simulink model "BitwiseAnd"  (R2014a)
settings: Solver=ode45  StartTime=0.0  StopTime=10.0  RelTol=1e-3
libraries: hdlsllib x17
settings Model: Creator=you.r  LastModifiedBy=you.r

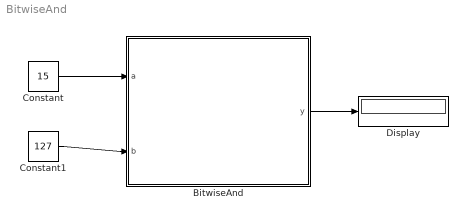
== system BitwiseAnd ==
  BitwiseAnd : Subsystem
  Constant : Constant  Value=15  OutDataTypeStr=uint8  SampleTime=1
  Constant1 : Constant  Value=127  OutDataTypeStr=uint8  SampleTime=-1
  Display : Display
  wires:
  Constant/1 -> BitwiseAnd/1(a)
  Constant1/1 -> BitwiseAnd/2(b)
  BitwiseAnd/1(y) -> Display/1

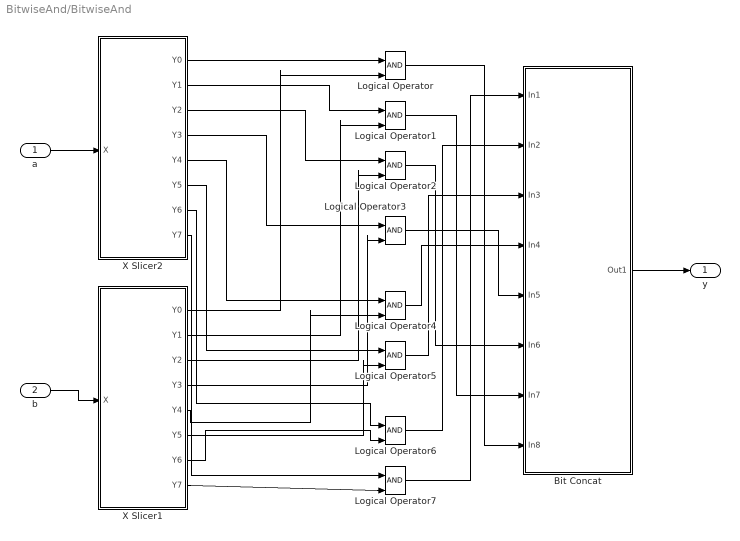
== system BitwiseAnd/BitwiseAnd ==
  a : Inport  OutDataTypeStr=uint8  SampleTime=1
  b : Inport  Port=2  OutDataTypeStr=uint8  SampleTime=1
  Bit Concat : Subsystem
  Logical Operator{,1..7} (8 alike) : Logic  IconShape=distinctive  AllPortsSameDT=off  OutDataTypeStr=boolean  SampleTime=1
  X Slicer1 : Subsystem
  X Slicer2 : Subsystem
  y : Outport  SampleTime=1
  wires:
  b/1 -> X Slicer1/1(X)
  a/1 -> X Slicer2/1(X)
  Logical Operator2/1 -> Bit Concat/6(In6)
  Logical Operator4/1 -> Bit Concat/4(In4)
  Logical Operator7/1 -> Bit Concat/1(In1)
  Logical Operator/1 -> Bit Concat/8(In8)
  Logical Operator1/1 -> Bit Concat/7(In7)
  Logical Operator6/1 -> Bit Concat/2(In2)
  Logical Operator5/1 -> Bit Concat/3(In3)
  Logical Operator3/1 -> Bit Concat/5(In5)
  X Slicer1/8(Y7) -> Logical Operator7/2
  X Slicer1/5(Y4) -> Logical Operator4/2
  X Slicer2/4(Y3) -> Logical Operator3/1
  X Slicer2/8(Y7) -> Logical Operator7/1
  X Slicer2/3(Y2) -> Logical Operator2/1
  X Slicer2/6(Y5) -> Logical Operator5/1
  X Slicer2/2(Y1) -> Logical Operator1/1
  X Slicer1/3(Y2) -> Logical Operator2/2
  X Slicer1/2(Y1) -> Logical Operator1/2
  X Slicer1/7(Y6) -> Logical Operator6/2
  X Slicer2/7(Y6) -> Logical Operator6/1
  X Slicer2/5(Y4) -> Logical Operator4/1
  X Slicer1/1(Y0) -> Logical Operator/2
  X Slicer2/1(Y0) -> Logical Operator/1
  X Slicer1/6(Y5) -> Logical Operator5/2
  X Slicer1/4(Y3) -> Logical Operator3/2
  Bit Concat/1(Out1) -> y/1

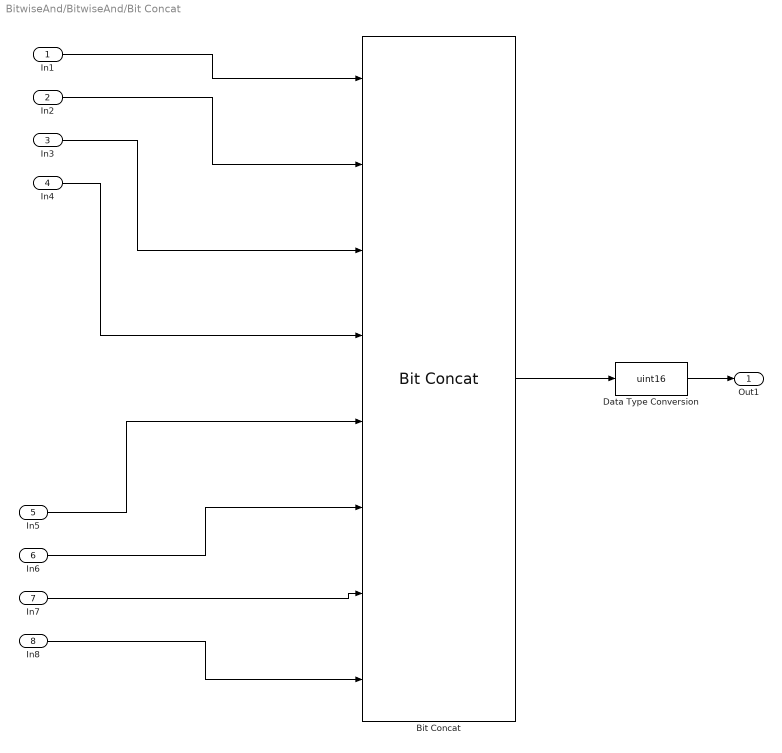
== system BitwiseAnd/BitwiseAnd/Bit Concat ==
  In1 : Inport
  In2 : Inport  Port=2
  In3 : Inport  Port=3
  In4 : Inport  Port=4
  In5 : Inport  Port=5
  In6 : Inport  Port=6
  In7 : Inport  Port=7
  In8 : Inport  Port=8
  Bit Concat : hdlsllib/HDL Operations/Bit Concat  numInputs=8
  Data Type Conversion : DataTypeConversion  OutDataTypeStr=uint16
  Out1 : Outport
  wires:
  Data Type Conversion/1 -> Out1/1
  Bit Concat/1 -> Data Type Conversion/1
  In7/1 -> Bit Concat/7
  In1/1 -> Bit Concat/1
  In8/1 -> Bit Concat/8
  In6/1 -> Bit Concat/6
  In2/1 -> Bit Concat/2
  In5/1 -> Bit Concat/5
  In3/1 -> Bit Concat/3
  In4/1 -> Bit Concat/4

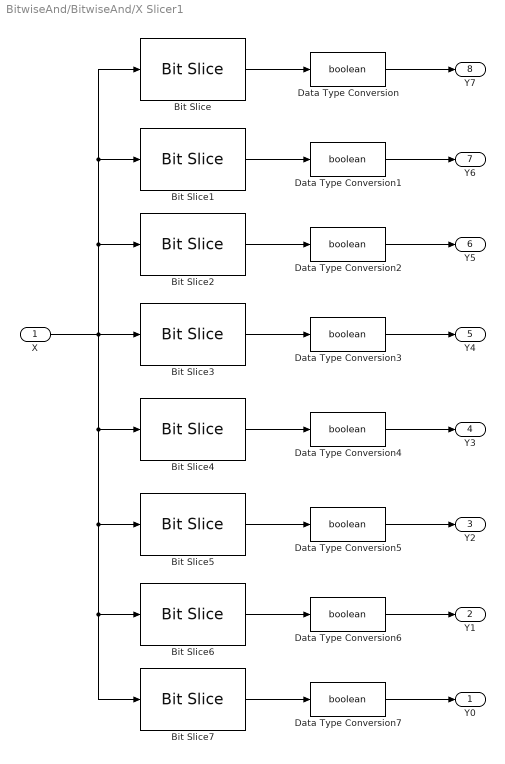
== system BitwiseAnd/BitwiseAnd/X Slicer1 ==
  X : Inport  OutDataTypeStr=uint8  SampleTime=1
  Bit Slice : hdlsllib/HDL Operations/Bit Slice  lidx=7  ridx=7
  Bit Slice1 : hdlsllib/HDL Operations/Bit Slice  lidx=6  ridx=6
  Bit Slice2 : hdlsllib/HDL Operations/Bit Slice  lidx=5  ridx=5
  Bit Slice3 : hdlsllib/HDL Operations/Bit Slice  lidx=4  ridx=4
  Bit Slice4 : hdlsllib/HDL Operations/Bit Slice  lidx=3  ridx=3
  Bit Slice5 : hdlsllib/HDL Operations/Bit Slice  lidx=2  ridx=2
  Bit Slice6 : hdlsllib/HDL Operations/Bit Slice  lidx=1  ridx=1
  Bit Slice7 : hdlsllib/HDL Operations/Bit Slice  lidx=0  ridx=0
  Data Type Conversion{,1..7} (8 alike) : DataTypeConversion  OutDataTypeStr=boolean
  Y0 : Outport  OutDataTypeStr=boolean  SampleTime=1
  Y1 : Outport  Port=2  OutDataTypeStr=boolean  SampleTime=1
  Y2 : Outport  Port=3  OutDataTypeStr=boolean  SampleTime=1
  Y3 : Outport  Port=4  OutDataTypeStr=boolean  SampleTime=1
  Y4 : Outport  Port=5  OutDataTypeStr=boolean  SampleTime=1
  Y5 : Outport  Port=6  OutDataTypeStr=boolean  SampleTime=1
  Y6 : Outport  Port=7  OutDataTypeStr=boolean  SampleTime=1
  Y7 : Outport  Port=8  OutDataTypeStr=boolean  SampleTime=1
  wires:
  X/1 -> Bit Slice4/1, Bit Slice5/1, Bit Slice6/1, Bit Slice7/1, Bit Slice3/1, Bit Slice2/1, Bit Slice1/1, Bit Slice/1
  Data Type Conversion/1 -> Y7/1
  Data Type Conversion1/1 -> Y6/1
  Bit Slice2/1 -> Data Type Conversion2/1
  Bit Slice3/1 -> Data Type Conversion3/1
  Bit Slice4/1 -> Data Type Conversion4/1
  Data Type Conversion6/1 -> Y1/1
  Bit Slice/1 -> Data Type Conversion/1
  Bit Slice1/1 -> Data Type Conversion1/1
  Bit Slice6/1 -> Data Type Conversion6/1
  Data Type Conversion7/1 -> Y0/1
  Bit Slice7/1 -> Data Type Conversion7/1
  Bit Slice5/1 -> Data Type Conversion5/1
  Data Type Conversion2/1 -> Y5/1
  Data Type Conversion3/1 -> Y4/1
  Data Type Conversion4/1 -> Y3/1
  Data Type Conversion5/1 -> Y2/1

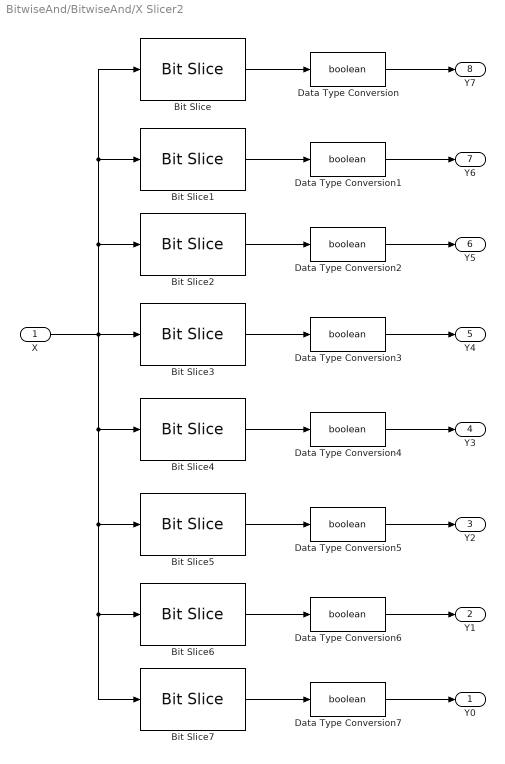
== system BitwiseAnd/BitwiseAnd/X Slicer2 ==
  X : Inport  OutDataTypeStr=uint8  SampleTime=1
  Bit Slice : hdlsllib/HDL Operations/Bit Slice  lidx=7  ridx=7
  Bit Slice1 : hdlsllib/HDL Operations/Bit Slice  lidx=6  ridx=6
  Bit Slice2 : hdlsllib/HDL Operations/Bit Slice  lidx=5  ridx=5
  Bit Slice3 : hdlsllib/HDL Operations/Bit Slice  lidx=4  ridx=4
  Bit Slice4 : hdlsllib/HDL Operations/Bit Slice  lidx=3  ridx=3
  Bit Slice5 : hdlsllib/HDL Operations/Bit Slice  lidx=2  ridx=2
  Bit Slice6 : hdlsllib/HDL Operations/Bit Slice  lidx=1  ridx=1
  Bit Slice7 : hdlsllib/HDL Operations/Bit Slice  lidx=0  ridx=0
  Data Type Conversion{,1..7} (8 alike) : DataTypeConversion  OutDataTypeStr=boolean
  Y0 : Outport  OutDataTypeStr=boolean  SampleTime=1
  Y1 : Outport  Port=2  OutDataTypeStr=boolean  SampleTime=1
  Y2 : Outport  Port=3  OutDataTypeStr=boolean  SampleTime=1
  Y3 : Outport  Port=4  OutDataTypeStr=boolean  SampleTime=1
  Y4 : Outport  Port=5  OutDataTypeStr=boolean  SampleTime=1
  Y5 : Outport  Port=6  OutDataTypeStr=boolean  SampleTime=1
  Y6 : Outport  Port=7  OutDataTypeStr=boolean  SampleTime=1
  Y7 : Outport  Port=8  OutDataTypeStr=boolean  SampleTime=1
  wires:
  X/1 -> Bit Slice4/1, Bit Slice5/1, Bit Slice6/1, Bit Slice7/1, Bit Slice3/1, Bit Slice2/1, Bit Slice1/1, Bit Slice/1
  Data Type Conversion/1 -> Y7/1
  Data Type Conversion1/1 -> Y6/1
  Bit Slice2/1 -> Data Type Conversion2/1
  Bit Slice3/1 -> Data Type Conversion3/1
  Bit Slice4/1 -> Data Type Conversion4/1
  Data Type Conversion6/1 -> Y1/1
  Bit Slice/1 -> Data Type Conversion/1
  Bit Slice1/1 -> Data Type Conversion1/1
  Bit Slice6/1 -> Data Type Conversion6/1
  Data Type Conversion7/1 -> Y0/1
  Bit Slice7/1 -> Data Type Conversion7/1
  Bit Slice5/1 -> Data Type Conversion5/1
  Data Type Conversion2/1 -> Y5/1
  Data Type Conversion3/1 -> Y4/1
  Data Type Conversion4/1 -> Y3/1
  Data Type Conversion5/1 -> Y2/1
